simulink model "sf_temp_logic"  (R2015b)
settings: Solver=ode45  StartTime=0.0  StopTime=20  RelTol=1e-3
libraries: simulink x1
settings Model: Creator=amatsumo  LastModifiedBy=amatsumo
settings DataIOCC: SaveFormat=Array
settings DebuggingCC: UnderspecifiedInitializationDetection=Classic  MergeDetectMultiDrivingBlocksExec=none  SolverPrmCheckMsg=warning  StateNameClashWarn=warning
settings HardwareCC: ProdBitPerPointer=32  ProdLargestAtomicFloat=None  ProdIntDivRoundTo=Undefined  ProdEndianess=Unspecified  ProdWordSize=32  ProdHWDeviceType=32-bit Generic
settings GRTTargetCC: GeneratePreprocessorConditionals=Disable all
settings ConfigComp: CovModelRefEnable=Off  CovSFcnEnable=off

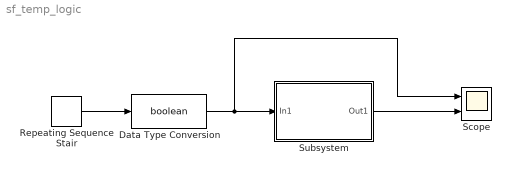
== system sf_temp_logic ==
  Data Type Conversion : DataTypeConversion  OutDataTypeStr=boolean
  Repeating Sequence Stair : simulink/Sources/Repeating Sequence Stair  OutValues=[0 1 1 zeros(1,4) 1 1 1 zeros(1,6)].'  tsamp=1  OutMin=[]  OutMax=[]  OutDataTypeStr=double  OutputDataTypeScalingMode=double  OutDataType=fixdt(0,8)  ConRadixGroup=Best Precision: Vector-wise  OutScaling=2^-12
  Scope : Scope  NumInputPorts=2
  Subsystem : Subsystem
  wires:
  Repeating Sequence Stair/1 -> Data Type Conversion/1
  Data Type Conversion/1 -> Subsystem/1(In1), Scope/1
  Subsystem/1(Out1) -> Scope/2

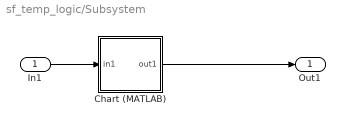
== system sf_temp_logic/Subsystem ==
  In1 : Inport
  Chart (MATLAB) : Stateflow chart  TreatAsAtomicUnit=on
  Out1 : Outport
  wires:
  In1/1 -> Chart (MATLAB)/1(in1)
  Chart (MATLAB)/1(out1) -> Out1/1

== stateflow chart sf_temp_logic/Subsystem/Chart (MATLAB) ==
  settings: stateMachineType=MOORE_MACHINE  initializeOutput=1
  state Init/
    out1 = fi(0,0,2,0);
  state On1/
    out1 = fi(1,0,2,0);
  state On2/
    out1 = fi(2,0,2,0);
  (default) -> Init
  Init -> On1 : [in1 > 0]
  On1 -> Init [order 2] : [in1 == 0]
  On1 -> On2 [order 1] : [after(3,tick)]
  On2 -> On1 : [after(4,tick)]
  data: in1 input boolean; out1 output fixdt(0,2,0)
